simulink model "profacc"  (R2025b)
settings: Solver=FixedStepAuto  StartTime=0.0  StopTime=inf  FixedStep=0.05  RelTol=1e-3
libraries: robotlib x8
settings Model: Creator=sprinkle  LastModifiedBy=sprinkle
settings OptimizationCC: DefaultParameterBehavior=Inlined  EnhancedBackFolding=on  PassReuseOutputArgsAs=Individual arguments  ZeroExternalMemoryAtStartup=off  ZeroInternalMemoryAtStartup=off  MaxStackSize=64  OptimizeBlockOrder=speed  DifferentSizesBufferReuse=on  OptimizationCustomize=off  EfficientTunableParamExpr=on
settings DebuggingCC: ParameterTunabilityLossMsg=error
settings HardwareCC: ProdBitPerPointer=32.0  ProdBitPerSizeT=32.0  ProdBitPerPtrDiffT=32.0  ProdLargestAtomicFloat=None  ProdIntDivRoundTo=Undefined  ProdEndianess=Unspecified  ProdWordSize=32.0  ProdHWDeviceType=Generic->Unspecified (assume 32-bit Generic)
settings SFSimCC: MATLABDynamicMemAlloc=off
settings RTWCC: SystemTargetFile=ert.tlc  HardwareBoard=Robot Operating System (ROS)  TLCOptions="-aInlineSetEventsForThisBaseRateFcn=TLC_FALSE -aSuppressMultiTaskScheduler=TLC_FALSE  -aRateBasedStepFcn=0"  GenCodeOnly=on  TemplateMakefile=ert_default_tmf  Toolchain=Catkin  TargetLang=C++  Description=Embedded Coder
settings CodeAppCC: ForceParamTrailComments=on  IgnoreCustomStorageClasses=off  OperatorAnnotations=on  SimulinkDataObjDesc=on  SFDataObjDesc=on  InsertBlockDesc=on

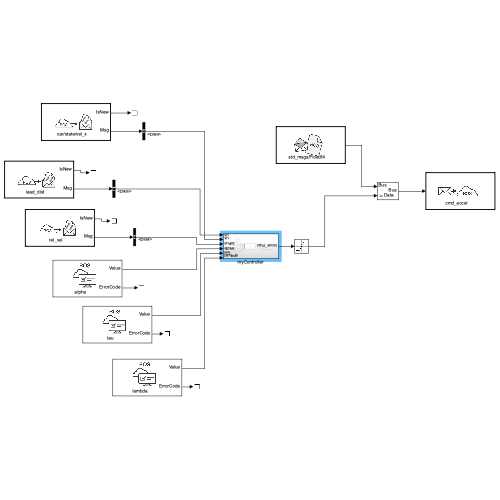
[thumbnail: Simulink's stored preview of the top-level diagram]
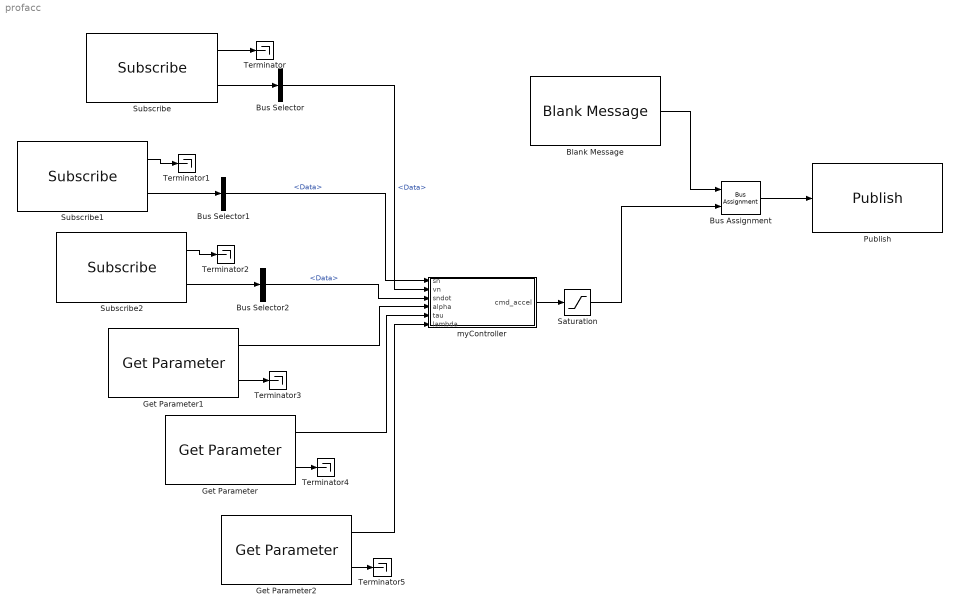
== system profacc ==
  Blank Message : robotlib/Blank Message  messageClass=Message  entityType=std_msgs/Float64  messageType=std_msgs/Float64  SampleTime=inf  legacyBusStruct=off
  Bus Assignment : BusAssignment  AssignedSignals=Data
  Bus Selector : BusSelector  OutputSignals=Data
  Bus Selector1 : BusSelector  OutputSignals=Data
  Bus Selector2 : BusSelector  OutputSignals=Data
  Get Parameter : robotlib/Get Parameter  ParameterSource=Specify your own  ParameterName=tau  ParameterType=double  ParameterMaxArrayLength=16  ParameterInitialValue=2.0  SampleTime=-1  ShowErrorCodeOutput=on  ModelName=profacc  BlockId=ParamGet_profacc_18
  Get Parameter1 : robotlib/Get Parameter  ParameterSource=Specify your own  ParameterName=alpha  ParameterType=double  ParameterMaxArrayLength=16  ParameterInitialValue=1.1  SampleTime=-1  ShowErrorCodeOutput=on  ModelName=profacc  BlockId=ParamGet_profacc_19
  Get Parameter2 : robotlib/Get Parameter  ParameterSource=Specify your own  ParameterName=lambda  ParameterType=double  ParameterMaxArrayLength=16  ParameterInitialValue=0.1  SampleTime=-1  ShowErrorCodeOutput=on  ModelName=profacc  BlockId=ParamGet_profacc_52
  Publish : robotlib/Publish  topicSource=Specify your own  topic=cmd_accel  messageType=std_msgs/Float64  legacyBusStruct=off  messageQueueLength=1
  Saturation : Saturate  UpperLimit=1.5  LowerLimit=-3.0
  Subscribe : robotlib/Subscribe  topicSource=Specify your own  topic=car/state/vel_x  messageType=std_msgs/Float64  SampleTime=-1  legacyBusStruct=off  messageQueueLength=1
  Subscribe1 : robotlib/Subscribe  topicSource=Specify your own  topic=lead_dist  messageType=std_msgs/Float64  SampleTime=-1  legacyBusStruct=off  messageQueueLength=1
  Subscribe2 : robotlib/Subscribe  topicSource=Specify your own  topic=rel_vel  messageType=std_msgs/Float64  SampleTime=-1  legacyBusStruct=off  messageQueueLength=1
  Terminator{,1..5} (6 alike) : Terminator
  myController : Subsystem
  wires:
  Subscribe/2 -> Bus Selector/1
  Subscribe/1 -> Terminator/1
  Subscribe1/1 -> Terminator1/1
  Blank Message/1 -> Bus Assignment/1
  Bus Assignment/1 -> Publish/1
  Bus Selector/1 -> myController/2(vn)  "<Data>"
  myController/1(cmd_accel) -> Saturation/1
  Get Parameter/1 -> myController/5(tau)
  Get Parameter1/1 -> myController/4(alpha)
  Saturation/1 -> Bus Assignment/2
  Subscribe1/2 -> Bus Selector1/1
  Bus Selector1/1 -> myController/1(sn)  "<Data>"
  Subscribe2/1 -> Terminator2/1
  Bus Selector2/1 -> myController/3(sndot)  "<Data>"
  Subscribe2/2 -> Bus Selector2/1
  Get Parameter1/2 -> Terminator3/1
  Get Parameter/2 -> Terminator4/1
  Get Parameter2/1 -> myController/6(lambda)
  Get Parameter2/2 -> Terminator5/1

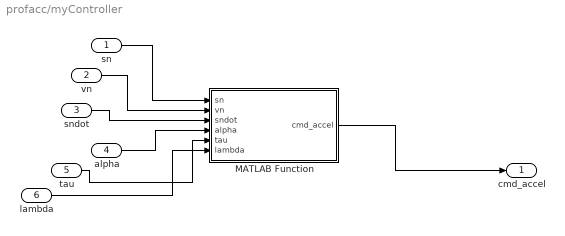
== system profacc/myController ==
  sn : Inport
  vn : Inport  Port=2
  sndot : Inport  Port=3
  alpha : Inport  Port=4
  tau : Inport  Port=5
  lambda : Inport  Port=6
  MATLAB Function : MATLAB Function  TreatAsAtomicUnit=on
  cmd_accel : Outport
  wires:
  MATLAB Function/1(cmd_accel) -> cmd_accel/1
  tau/1 -> MATLAB Function/5(tau)
  alpha/1 -> MATLAB Function/4(alpha)
  sn/1 -> MATLAB Function/1(sn)
  vn/1 -> MATLAB Function/2(vn)
  sndot/1 -> MATLAB Function/3(sndot)
  lambda/1 -> MATLAB Function/6(lambda)

== matlab function profacc/myController/MATLAB Function ==
  data: sn input; cmd_accel output; vn input; sndot input; alpha input; tau input; lambda input
function cmd_accel = fcn(sn,vn,sndot,alpha,tau,lambda)

cmd_accel = alpha * (sn - tau*vn + lambda*sndot);
